simulink model "try_20260318"  (R2025b)
settings: Solver=FixedStepAuto  StartTime=0.0  StopTime=10.0  FixedStep=0.01  RelTol=1e-3
libraries: simulink x1
settings Model: Creator=itsyu  LastModifiedBy=itsyu

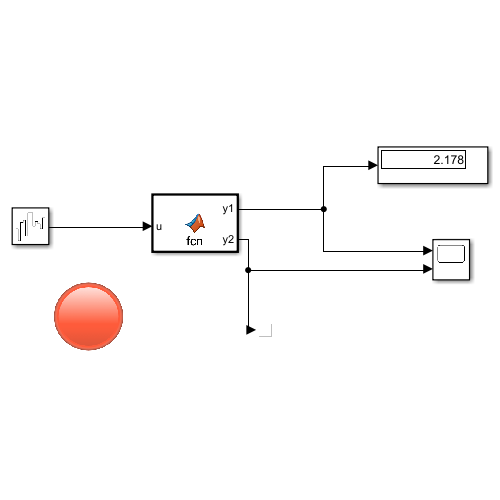
[thumbnail: Simulink's stored preview of the top-level diagram]
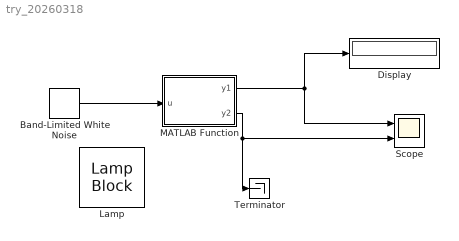
== system try_20260318 ==
  Band-Limited White Noise : simulink/Sources/Band-Limited White Noise  Cov=[0.1]  Ts=0.1  seed=[23341]
  Display : Display
  Lamp : LampBlock  LabelPosition=Hide  DefaultColor=[192.0, 192.0, 192.0]
  MATLAB Function : MATLAB Function  TreatAsAtomicUnit=on
  Scope : Scope  NumInputPorts=2
      settings: ActiveDisplayYMinimum=-0.5705718993485438  ActiveDisplayYMaximum=4.193617172130697
  Terminator : Terminator
  wires:
  Band-Limited White Noise/1 -> MATLAB Function/1(u)
  MATLAB Function/1(y1) -> Scope/1, Display/1
  MATLAB Function/2(y2) -> Scope/2, Terminator/1

== matlab function try_20260318/MATLAB Function ==
  data: u input; y1 output; y2 output
function [y1,y2] = fcn(u)

% if u > 0
%     y2 = 1;
% else
%     y2 = 0;
% end

% y1 = u;
 [y1, y2] = tryMe(u);

end
